simulink model "ETC_sim"  (R2023a)
settings: Solver=ode45  StartTime=0.0  StopTime=20.0  RelTol=1e-3  EnableMultiTasking=on
PreLoadFcn:
  | J = 2.45e-4;
  | Vrise = 0.6;
  | Vdrop = 0.0;
  | Vfree = 1.83;
  | Vclose  = 0.5;
  | Vopen = 4.5;
  | Kp = 0.3;
  | Ki = 2.0;
  | Ts = .01;
libraries: simulink x1
settings Model: ParamWorkspaceSource=ReferencedWorkspace  Creator=nicholas  LastModifiedBy=Boss
settings SolverCC: AlgebraicLoopSolver=TrustRegion
settings DataIOCC: LimitDataPoints=on  SaveFormat=Array  SignalLoggingSaveFormat=ModelDataLogs  ReturnWorkspaceOutputs=off  SignalLoggingName=sigsOut
settings OptimizationCC: ExpressionDepthLimit=2147483647  InitFltsAndDblsToZero=on  LifeSpan=inf
settings DebuggingCC: SaveWithParameterizedLinksMsg=none  UnderspecifiedInitializationDetection=Classic  MergeDetectMultiDrivingBlocksExec=none  SignalResolutionControl=TryResolveAllWithWarning  MultiTaskDSMMsg=warning  MultiTaskCondExecSysMsg=none  FcnCallInpInsideContextMsg=warning  UnconnectedInputMsg=warning  UnconnectedOutputMsg=warning  UnconnectedLineMsg=warning  StateNameClashWarn=warning  SFUnexpectedBacktrackingDiag=warning  SFNoUnconditionalDefaultTransitionDiag=warning  SFExecutionAtInitializationDiag=none  ArithmeticOperatorsInVariantConditions=warning
settings HardwareCC: ProdBitPerPointer=32  ProdBitPerSizeT=32  ProdBitPerPtrDiffT=32  ProdLargestAtomicFloat=None  ProdIntDivRoundTo=Undefined  ProdEndianess=Unspecified  ProdWordSize=32  ProdHWDeviceType=32-bit Generic  TargetIntDivRoundTo=Zero  TargetEndianess=BigEndian  TargetHWDeviceType=Motorola PowerPC
settings ModelReferenceCC: PropagateSignalLabelsOutOfModel=off
settings CodeAppCC: StateflowObjectComments=on
settings GRTTargetCC: TargetFcnLib=ansi_tfl_tmw.mat  TargetLangStandard=C89/C90 (ANSI)  CombineOutputUpdateFcns=off  GRTInterface=on
settings ConfigComp: CovMetricSettings=dw  CovSaveCumulativeToWorkspaceVar=on  CovSaveSingleToWorkspaceVar=on

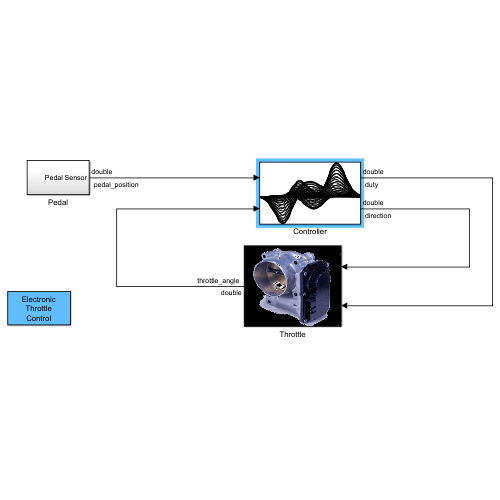
[thumbnail: Simulink's stored preview of the top-level diagram]
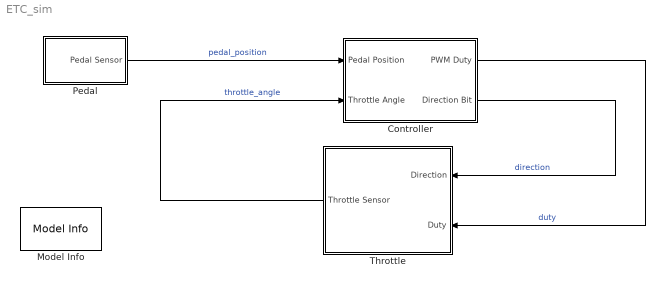
== system ETC_sim ==
  Controller : Subsystem
      mask Display: plot(peaks)
  Model Info : simulink/Model-Wide Utilities/Model Info  Frame=on  DisplayStringWithTags=|  HorizontalTextAlignment=Center  LeftAlignmentValue=0.5
      | Electronic
      | Throttle
      | Control
  Pedal : Subsystem
  Throttle : Subsystem
      mask Display: image(imread('throttle.png'))
  wires:
  Throttle/1(Throttle Sensor) -> Controller/2(Throttle Angle)  "throttle_angle"
  Controller/1(PWM Duty) -> Throttle/2(Duty)  "duty"
  Controller/2(Direction Bit) -> Throttle/1(Direction)  "direction"
  Pedal/1(Pedal Sensor) -> Controller/1(Pedal Position)  "pedal_position"

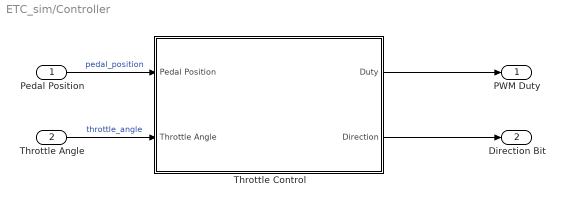
== system ETC_sim/Controller ==
  Pedal Position : Inport
  Throttle Angle : Inport  Port=2
  Throttle Control : Subsystem
  PWM Duty : Outport
  Direction Bit : Outport  Port=2
  wires:
  Throttle Control/1(Duty) -> PWM Duty/1
  Throttle Control/2(Direction) -> Direction Bit/1
  Throttle Angle/1 -> Throttle Control/2(Throttle Angle)  "throttle_angle"
  Pedal Position/1 -> Throttle Control/1(Pedal Position)  "pedal_position"

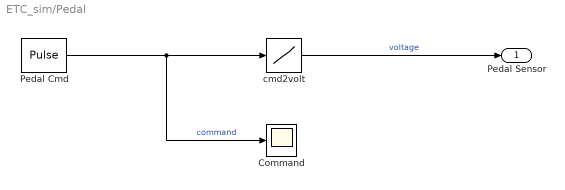
== system ETC_sim/Pedal ==
  Command : Scope
  Pedal Cmd : DiscretePulseGenerator  PulseType=Time based  Amplitude=0.9  Period=10  PulseWidth=50  PhaseDelay=2.5
  cmd2volt : Lookup  InputValues=[0 1]  Table=[Vrise Vdrop]  LookUpMeth=Interpolation-Use End Values  SaturateOnIntegerOverflow=off
  Pedal Sensor : Outport
  wires:
  Pedal Cmd/1 -> cmd2volt/1, Command/1  "command"
  cmd2volt/1 -> Pedal Sensor/1  "voltage"

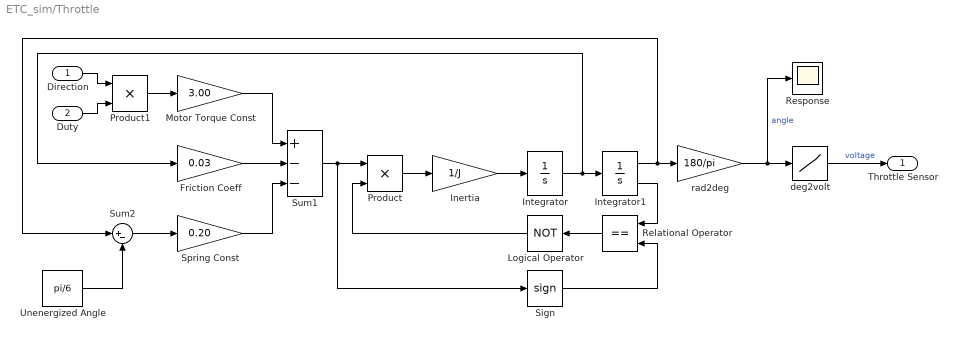
== system ETC_sim/Throttle ==
  Direction : Inport
  Duty : Inport  Port=2
  Friction Coeff : Gain  Gain=0.03  SaturateOnIntegerOverflow=on  OutDataTypeStr=Inherit: Same as input  ParamDataTypeStr=Inherit: Same as input
  Inertia : Gain  Gain=1/J  SaturateOnIntegerOverflow=on  OutDataTypeStr=Inherit: Same as input  ParamDataTypeStr=Inherit: Same as input
  Integrator : Integrator
  Integrator1 : Integrator  InitialCondition=pi/6  LimitOutput=on  UpperSaturationLimit=pi/2  LowerSaturationLimit=0  ShowSaturationPort=on
      settings: AttributesFormatString=%<LowerSaturationLimit> < th < %<UpperSaturationLimit>
  Logical Operator : Logic  Operator=NOT  AllPortsSameDT=off
  Motor Torque Const : Gain  Gain=3.00  SaturateOnIntegerOverflow=on  OutDataTypeStr=Inherit: Same as input  ParamDataTypeStr=Inherit: Same as input
  Product : Product  SaturateOnIntegerOverflow=on  OutDataTypeStr=Inherit: Same as first input
  Product1 : Product  SaturateOnIntegerOverflow=on  OutDataTypeStr=Inherit: Same as first input
  Relational Operator : RelationalOperator  Operator===  InputSameDT=off
  Response : Scope
  Sign : Signum
  Spring Const : Gain  Gain=0.20  SaturateOnIntegerOverflow=on  OutDataTypeStr=Inherit: Same as input  ParamDataTypeStr=Inherit: Same as input
  Sum1 : Sum  Inputs=+--  SaturateOnIntegerOverflow=on
  Sum2 : Sum  Inputs=|+-  SaturateOnIntegerOverflow=on
  Unenergized Angle : Constant  Value=pi/6
  deg2volt : Lookup  InputValues=[0 90]  Table=[Vclose Vopen]  LookUpMeth=Interpolation-Use End Values  OutDataTypeStr=double  SaturateOnIntegerOverflow=off
  rad2deg : Gain  Gain=180/pi  SaturateOnIntegerOverflow=on  OutDataTypeStr=Inherit: Same as input  ParamDataTypeStr=Inherit: Same as input
  Throttle Sensor : Outport
  wires:
  Product1/1 -> Motor Torque Const/1
  rad2deg/1 -> deg2volt/1, Response/1  "angle"
  Logical Operator/1 -> Product/2
  Relational Operator/1 -> Logical Operator/1
  Sign/1 -> Relational Operator/2
  Product/1 -> Inertia/1
  Unenergized Angle/1 -> Sum2/2
  Sum2/1 -> Spring Const/1
  Integrator1/2 -> Relational Operator/1
  Integrator1/1 -> Sum2/1, rad2deg/1
  Integrator/1 -> Friction Coeff/1, Integrator1/1
  Inertia/1 -> Integrator/1
  deg2volt/1 -> Throttle Sensor/1  "voltage"
  Sum1/1 -> Product/1, Sign/1
  Direction/1 -> Product1/1
  Duty/1 -> Product1/2
  Spring Const/1 -> Sum1/3
  Motor Torque Const/1 -> Sum1/1
  Friction Coeff/1 -> Sum1/2

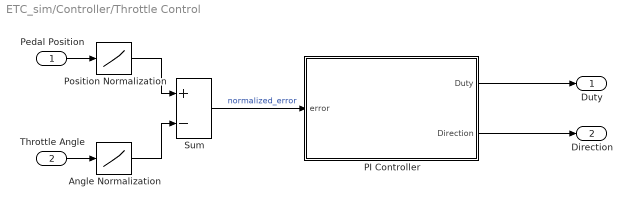
== system ETC_sim/Controller/Throttle Control ==
  Pedal Position : Inport
  Throttle Angle : Inport  Port=2
  Angle Normalization : Lookup  InputValues=[Vfree Vopen]  Table=[0 1]  LookUpMeth=Interpolation-Use End Values  OutDataTypeStr=double  SaturateOnIntegerOverflow=off
  PI Controller : Subsystem
  Position Normalization : Lookup  InputValues=[Vdrop Vrise]  Table=[1 0]  LookUpMeth=Interpolation-Use End Values  OutDataTypeStr=double  SaturateOnIntegerOverflow=off
  Sum : Sum  Inputs=+-
  Duty : Outport
  Direction : Outport  Port=2
  wires:
  Pedal Position/1 -> Position Normalization/1
  Throttle Angle/1 -> Angle Normalization/1
  PI Controller/1(Duty) -> Duty/1
  Sum/1 -> PI Controller/1(error)  "normalized_error"
  Angle Normalization/1 -> Sum/2
  Position Normalization/1 -> Sum/1
  PI Controller/2(Direction) -> Direction/1

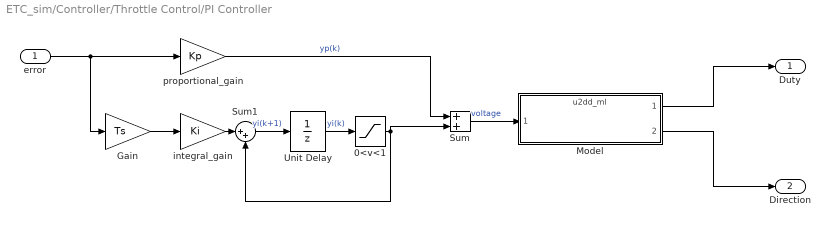
== system ETC_sim/Controller/Throttle Control/PI Controller ==
  error : Inport  SampleTime=Ts
  0<v<1 : Saturate  UpperLimit=1  LowerLimit=0
  Gain : Gain  Gain=Ts  SaturateOnIntegerOverflow=on  OutDataTypeStr=Inherit: Same as input  ParamDataTypeStr=Inherit: Same as input
  Model : ModelReference  ModelNameDialog=u2dd_ml.slx  SimulationMode=Normal  ModelReferenceVersion=1.3
  Sum : Sum  InputSameDT=on  SaturateOnIntegerOverflow=on  OutDataTypeStr=Inherit: Same as first input
  Sum1 : Sum  Inputs=|++  InputSameDT=on  SaturateOnIntegerOverflow=on  OutDataTypeStr=Inherit: Same as first input
  Unit Delay : UnitDelay  SampleTime=.01
      settings: AttributesFormatString=yi0 = %<X0>\n\n
  integral_gain : Gain  Gain=Ki  SaturateOnIntegerOverflow=on  OutDataTypeStr=Inherit: Same as input  ParamDataTypeStr=Inherit: Same as input
  proportional_gain : Gain  Gain=Kp  SaturateOnIntegerOverflow=on  OutDataTypeStr=Inherit: Same as input  ParamDataTypeStr=Inherit: Same as input
  Duty : Outport
  Direction : Outport  Port=2
  wires:
  Model/1 -> Duty/1
  Model/2 -> Direction/1
  proportional_gain/1 -> Sum/1  "yp(k)"
  error/1 -> proportional_gain/1, Gain/1
  integral_gain/1 -> Sum1/1
  Gain/1 -> integral_gain/1
  Unit Delay/1 -> 0<v<1/1  "yi(k)"
  Sum1/1 -> Unit Delay/1  "yi(k+1)"
  Sum/1 -> Model/1  "voltage"
  0<v<1/1 -> Sum/2, Sum1/2
